simulink model "car_controller2222"  (R2022a)
settings: Solver=ode1be  StartTime=0.0  StopTime=1000  FixedStep=0.005  RelTol=1e-4  AbsTol=1e-4
libraries: simulink_extras x3, sim3dlib x1, uavsim3dlib x1
settings Model: Creator=Sebas  LastModifiedBy=maxpr
settings SolverCC: AutoScaleAbsTol=off  SolverJacobianMethodControl=SparsePerturbation  ZeroCrossControl=EnableAll  EnableFixedStepZeroCrossing=on
settings DebuggingCC: AlgebraicLoopMsg=none  UnconnectedInputMsg=warning  UnconnectedOutputMsg=warning  UnconnectedLineMsg=warning

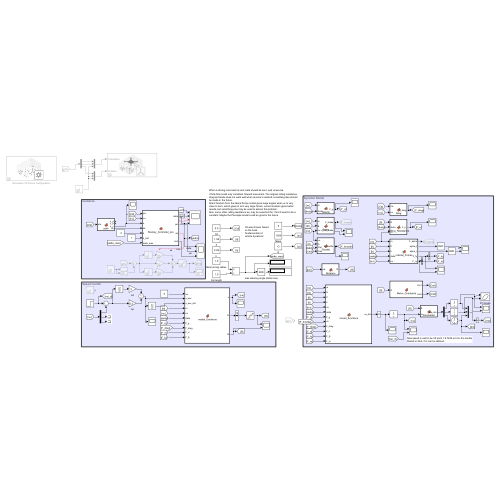
[thumbnail: Simulink's stored preview of the top-level diagram]
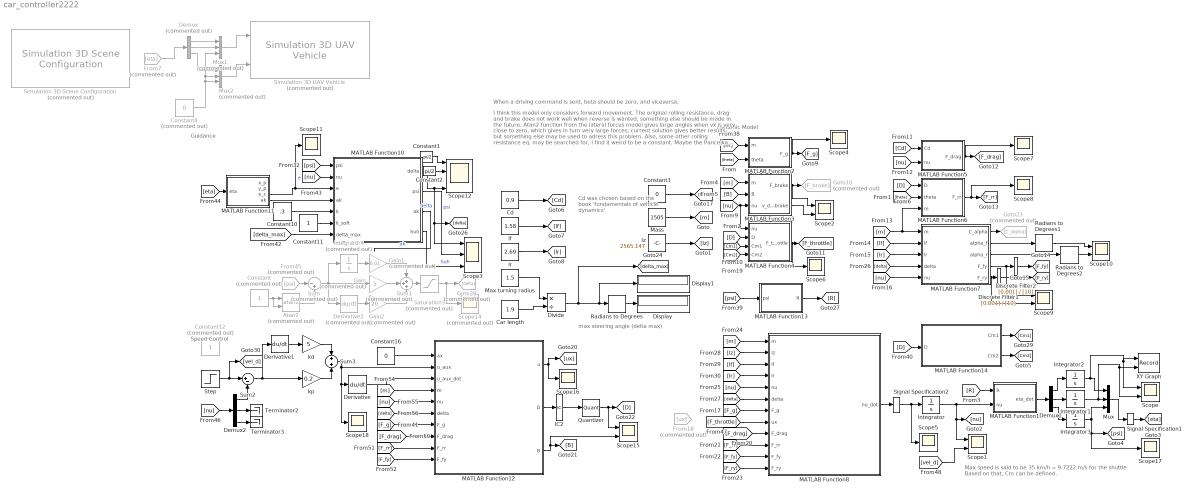
== system car_controller2222 ==
  note: Dynamic Model
  note: Guidance
  note: I think this model only considers forward movement. The original rolling resistance, drag and brake does not work well when reverse is wanted; something else should be made in the future.
      | Atan2 function from the lateral forces model gives large angles when vx is very close to zero, which gives in turn very large forces; current solution gives better results, but something else may be used to adress this problem.
      | Also, some other rolling resistance eq. may be searched for, I find it weird to be a constant. Maybe the Pancejka model could be good in the future.
  note: Max speed is said to be 35 km/h = 9.7222 m/s for the shuttle
      | Based on that, Cm can be defined.
  note: Cd was chosen based on the book 'fundamentals of vehicle dynamics'
  note: When a driving command is sent, beta should be zero, and viceversa.
  note: max steering angle (delta max)
  note: Speed Control
  Atan2 : Trigonometry  Commented=on  Operator=atan2
  Car length : Constant  Value=1.9
  Cd : Constant  Value=0.9
  Constant : Constant  Commented=on
  Constant1 : Constant  Value=-pi/2
  Constant10 : Constant  Value=.3
  Constant11 : Constant
  Constant12 : Constant  Commented=on
  Constant16 : Constant  Value=0
  Constant2 : Constant  Value=pi/2
  Constant3 : Constant  Value=0
  Constant4 : Constant  Commented=on  Value=0
  Demux : Demux  Commented=on  Outputs=3
  Demux1 : Demux  Outputs=3
  Demux2 : Demux  Outputs=3
  Derivative : Derivative
  Derivative1 : Derivative
  Derivative2 : Derivative  Commented=on
  Discrete Filter1 : DiscreteFilter  Numerator=[0.001]  Denominator=[10]
  Discrete Filter2 : DiscreteFilter  Numerator=[0.001]  Denominator=[10]
  Display : Display
  Display1 : Display
  Divide : Product  Inputs=*/
  From18 : From  Commented=on  GotoTag=ux
  From45 : From  Commented=on  GotoTag=psi
  From7 : From  Commented=on  GotoTag=eta
  Gain : Gain  Commented=on  Gain=5
  Gain1 : Gain  Commented=on  Gain=0.01
  Gain2 : Gain  Commented=on  Gain=20
  Goto10 : Goto  Commented=on  GotoTag=F_brake
  Goto23 : Goto  Commented=on  GotoTag=C_alpha
  Goto28 : Goto  Commented=on  GotoTag=delta
  IC2 : InitialCondition  Value=0
  Integrator : Integrator
  Integrator1 : Integrator
  Integrator2 : Integrator
  Integrator3 : Integrator  WrapState=on
  Integrator4 : Integrator  Commented=on
  Iz : Constant  Value=2565.147
  MATLAB Function1 : MATLAB Function  TreatAsAtomicUnit=on
  MATLAB Function10 : MATLAB Function  TreatAsAtomicUnit=on
  MATLAB Function11 : MATLAB Function  TreatAsAtomicUnit=on
  MATLAB Function12 : MATLAB Function  TreatAsAtomicUnit=on
  MATLAB Function13 : MATLAB Function  TreatAsAtomicUnit=on
  MATLAB Function14 : MATLAB Function  TreatAsAtomicUnit=on
  MATLAB Function2 : MATLAB Function  TreatAsAtomicUnit=on
  MATLAB Function3 : MATLAB Function  TreatAsAtomicUnit=on
  MATLAB Function4 : MATLAB Function  TreatAsAtomicUnit=on
  MATLAB Function5 : MATLAB Function  TreatAsAtomicUnit=on
  MATLAB Function6 : MATLAB Function  TreatAsAtomicUnit=on
  MATLAB Function7 : MATLAB Function  TreatAsAtomicUnit=on
  MATLAB Function8 : MATLAB Function  TreatAsAtomicUnit=on
  Mass : Constant  Value=1505
  Max turning radius : Constant  Value=1.5
  Mux : Mux  Inputs=3
  Mux1 : Mux  Commented=on  Inputs=3
  Mux2 : Mux  Commented=on  Inputs=3
  Quantizer : Quantizer  QuantizationInterval=1
  Radians to Degrees : simulink_extras/Transformations/Radians to Degrees
  Radians to Degrees1 : simulink_extras/Transformations/Radians to Degrees
  Radians to Degrees2 : simulink_extras/Transformations/Radians to Degrees
  Saturation3 : Saturate  Commented=on  UpperLimit=1.054  LowerLimit=-1.054
  Scope{,1..2,9..10,15} (6 alike) : Scope  NumInputPorts=2
  Scope{4..8,11,16..18} (9 alike) : Scope
  Scope12 : Scope  NumInputPorts=4
  Scope14 : Scope  Commented=on
  Scope3 : Scope  NumInputPorts=3
  Signal Specification1 : SignalSpecification
  Signal Specification2 : SignalSpecification  Dimensions=3
  Simulation 3D Scene Configuration : sim3dlib/Simulation 3D Scene Configuration  Priority=0  Commented=on  ProjectFormat=Default Scenes  SceneDesc=US city block  ProjectName=C:\Program Files\MATLAB\R2023a\toolbox\shared\sim3d_projects\automotive_project\UE4\WindowsNoEditor\VehicleSimulation.exe  ScenePath=/Game/Maps/USCityBlock  EnableOpenDRIVE=off  vehTagList={'Scene Origin';'SimulinkVehicle1'}  vehTag=Scene Origin  OpVisEn=off  Ts=.01  EnableWindow=on  EnableRemoteAccess=off  EnableWeather=off  SunAltitude=40.0  SunAzimuth=90  clouds=10  wind=1  fog=0  rain=0  sensorTag=MainCamera1  sensorId=1  sensorName=MainCamera1  mountLoc=Origin  offsetFlag=off  tmountOffset=[0, 0, 0]  rmountOffset=[0, 0, 0]  HorizontalResolution=1280  VerticalResolution=720  HorizontalFOV=60  mountPoint=[0 0 0]  mountOrientation=[0 0 0]  aMode=4  ID=1  GeoTrigger=Inactive
  Simulation 3D UAV Vehicle : uavsim3dlib/Simulation 3D UAV Vehicle  Priority=-1  Commented=on  Mesh=Quadrotor  MeshPath=/MathWorksUAVContent/UAVs/HexaRotorUAV/HexaRotor.HexaRotor  Color=Black  ActorName=SimulinkVehicle1  UseGlobalFrame=off  InitialTranslation=[0 0 0]  InitialRotation=[0 0 0]  InitialTranslationGlobal=[0 0 0]  InitialGeoOrigin=[0 0 0]  InitialRotationGlobal=[0 0 0]  SampleTime=-1  ActorType=SimulinkVehicle  ID=1  aMode=4  ActorTag=SimulinkVehicle1
  Step : Step  Time=0  Before=.5  After=.5  SampleTime=0
  Sum : Sum  Commented=on  Inputs=|-+
  Sum1 : Sum  Commented=on  Inputs=+++
  Sum2 : Sum  Inputs=|+-
  Sum3 : Sum
  Terminator2 : Terminator
  Terminator3 : Terminator
  XY Graph : Record  FileSettingsInternal="{\"entries\":[{\"content\":{\"excelSettings\":{\"content\":{},\"type\":\"Streamout.ExcelSettings\"}},\"type\":\"Streamout.FileSettingStorage\",\"uuid\":\"\"}],\"packageUris\":[\"http:\\/\\/schema.mathworks.com\\/mf0\\/streamout_blocks\\/R2020a\"],\"version\":\"1.0\"}"  Layout=[1 1]  SignalsInternal="{\"entries\":[{\"content\":{\"signals\":[{\"content\":{\"blockPath\":[],\"dimensions\":[1],\"domain\":\"\",\"lineColor\":\"#edb120\",\"plots\":[1],\"port\":1,\"signalID\":1411,\"signalName\":\"Integrator2\"},\"type\":\"RecordBlkView.Signal\",\"uuid\":\"\"},{\"content\":{\"blockPath\":[],\"dimensions\":[1],\"domain\":\"\",\"lineColor\":\"#7e2f8e\",\"plots\":[1],\"port\":2,\"signalID\":1414,\"signalName\":\"Integrator1\"},\"type\":\"RecordBlkView.Signal\",\"uuid\":\"\"}]},\"type\":\"RecordBlkView.InputSignals\",\"uuid\":\"\"}],\"packageUris\":[\"http:\\/\\/schema.mathworks.com\\/mf0\\/streamout_blocks\\/R2020a\"],\"version\":\"1.0\"}"  VisualizationBindings="{\"xyplotplugin\":{\"info\":[{\"series\":[{\"bindingParametersList\":[{\"parameter\":\"X-Axis\",\"signalID\":1411,\"signalName\":\"Integrator2\"},{\"parameter\":\"Y-Axis\",\"signalID\":1414,\"signalName\":\"Integrator1\"}],\"seriesID\":36310}],\"subplotID\":1}]}}"  CompatibilityTag=XY
  kd : Gain  Gain=5
  kp : Gain  Gain=0.2
  lf : Constant  Value=1.58
  lr : Constant  Value=2.69
  wires:
  Max turning radius/1 -> Divide/1
  Car length/1 -> Divide/2
  Radians to Degrees/1 -> Display/1
  Divide/1 -> Display1/1, Radians to Degrees/1, [delta_max]
  Iz/1 -> [Iz]
  Mass/1 -> [m]
  Cd/1 -> [Cd]
  lr/1 -> [lr]
  lf/1 -> [lf]
  [theta] -> MATLAB Function2/2(theta)
  [m] -> MATLAB Function3/1(m)
  [nu] -> MATLAB Function4/1(nu), MATLAB Function3/3(nu)
  [Cd] -> MATLAB Function5/1(Cd)
  [nu] -> MATLAB Function5/2(nu)
  [lf] -> MATLAB Function7/2(lf)
  [lr] -> MATLAB Function7/3(lr)
  [delta] -> MATLAB Function7/4(delta)
  [nu] -> MATLAB Function7/5(nu)
  MATLAB Function2/1(F_g) -> Scope4/1, [F_g]
  MATLAB Function3/1(F_brake) -> Scope2/1, Goto10/1
  MATLAB Function4/1(F_throttle) -> Scope6/1, [F_throttle]
  MATLAB Function5/1(F_drag) -> Scope7/1, [F_drag]
  MATLAB Function6/1(F_rr) -> Scope8/1, [F_rr]
  [F_g] -> MATLAB Function8/7(F_g)
  [F_drag] -> MATLAB Function8/9(F_drag)
  [F_rr] -> MATLAB Function8/10(F_rr)
  [F_fy] -> MATLAB Function8/11(F_fy)
  [F_ry] -> MATLAB Function8/12(F_ry)
  [m] -> MATLAB Function8/1(m)
  [nu] -> MATLAB Function8/5(nu)
  [delta] -> MATLAB Function8/6(delta)
  [Iz] -> MATLAB Function8/2(Iz)
  [lf] -> MATLAB Function8/3(lf)
  [lr] -> MATLAB Function8/4(lr)
  Integrator3/1 -> Scope17/1, [psi], Mux/3
  Demux1/3 -> Integrator3/1
  Integrator1/1 -> Scope/2, XY Graph/2, Mux/2
  Mux/1 -> Signal Specification1/1
  [R] -> MATLAB Function1/1(R)
  MATLAB Function1/1(eta_dot) -> Demux1/1
  Integrator/1 -> MATLAB Function1/2(nu), [nu], Scope1/1
  Integrator2/1 -> Scope/1, XY Graph/1, Mux/1
  Demux1/1 -> Integrator2/1
  Demux1/2 -> Integrator1/1
  [m] -> MATLAB Function2/1(m)
  [B] -> MATLAB Function3/2(B)
  MATLAB Function3/2(v_dot_brake) -> Scope2/2
  [m] -> MATLAB Function6/3(m), MATLAB Function7/1(m)
  Constant3/1 -> [theta]
  [theta] -> MATLAB Function6/2(theta)
  [D] -> MATLAB Function4/2(D)
  MATLAB Function7/3(alpha_r) -> Radians to Degrees2/1
  Radians to Degrees1/1 -> Scope10/1
  Radians to Degrees2/1 -> Scope10/2
  MATLAB Function7/1(C_alpha) -> Goto23/1
  Signal Specification1/1 -> [eta]
  MATLAB Function10/1(delta) -> Scope12/4, Scope3/1, [delta]  "delta"
  [eta] -> MATLAB Function11/1(eta)
  [psi] -> MATLAB Function10/1("psi ")
  MATLAB Function11/3(e_c) -> Scope11/1, MATLAB Function10/3(e)  "e"
  [nu] -> MATLAB Function10/2(nu)
  [delta_max] -> MATLAB Function10/7(delta_max)
  Constant11/1 -> MATLAB Function10/6(k_soft)
  Constant10/1 -> MATLAB Function10/5(k)
  Signal Specification2/1 -> Scope5/1, Integrator/1
  MATLAB Function7/2(alpha_f) -> Radians to Degrees1/1
  MATLAB Function7/5(F_ry) -> Scope9/2, Discrete Filter1/1
  MATLAB Function7/4(F_fy) -> Discrete Filter2/1, Scope9/1
  Discrete Filter1/1 -> [F_ry]
  Discrete Filter2/1 -> [F_fy]
  [psi] -> MATLAB Function13/1(psi)
  MATLAB Function13/1(R) -> [R]
  kp/1 -> Sum3/2
  Sum2/1 -> Derivative1/1, kp/1
  Demux2/1 -> Sum2/2
  Demux2/3 -> Terminator3/1
  Step/1 -> [vel_d], Sum2/1
  [nu] -> Demux2/1
  kd/1 -> Sum3/1
  Demux2/2 -> Terminator2/1
  Derivative1/1 -> kd/1
  Sum3/1 -> Scope18/1, Derivative/1, MATLAB Function12/2(u_aux)
  Constant16/1 -> MATLAB Function12/1(ax)
  MATLAB Function8/1(nu_dot) -> Signal Specification2/1
  [delta] -> MATLAB Function12/6(delta)
  [nu] -> MATLAB Function12/5(nu)
  [m] -> MATLAB Function12/4(m)
  [F_fy] -> MATLAB Function12/10(F_fy)
  [F_rr] -> MATLAB Function12/9(F_rr)
  [F_drag] -> MATLAB Function12/8(F_drag)
  [F_g] -> MATLAB Function12/7(F_g)
  MATLAB Function12/1(u) -> [ux], Scope16/1
  [F_throttle] -> MATLAB Function8/8(ux)
  Atan2/1 -> Sum/2
  Sum/1 -> Integrator4/1, Derivative2/1, Gain/1
  From45/1 -> Sum/1
  MATLAB Function12/3(B) -> Scope15/2, [B]
  MATLAB Function12/2(D) -> IC2/1
  Saturation3/1 -> Scope14/1, Goto28/1
  Sum1/1 -> Saturation3/1
  Derivative2/1 -> Gain2/1
  Constant/1 -> Atan2/2, Atan2/1
  Gain2/1 -> Sum1/3
  Gain/1 -> Sum1/2
  Integrator4/1 -> Gain1/1
  Gain1/1 -> Sum1/1
  Derivative/1 -> MATLAB Function12/3(u_aux_dot)
  MATLAB Function11/4(ak) -> MATLAB Function10/4("ak ")
  [D] -> MATLAB Function6/1(D)
  [Cm1] -> MATLAB Function4/3(Cm1)
  [Cm2] -> MATLAB Function4/4(Cm2)
  MATLAB Function14/2(Cm2) -> [Cm2]
  MATLAB Function14/1(Cm1) -> [Cm1]
  [D] -> MATLAB Function14/1(D)
  IC2/1 -> Quantizer/1
  Quantizer/1 -> Scope15/1, [D]
  [vel_d] -> Scope1/2
  Constant1/1 -> Scope12/1
  Constant2/1 -> Scope12/2
  ? -> Scope12/3
  MATLAB Function10/3(ak) -> ?  "ak"
  MATLAB Function10/2(psi) -> Scope3/2  "psi"
  MATLAB Function10/4(huh) -> Scope3/3  "huh"
  From7/1 -> Demux/1
  Demux/1 -> Mux1/1
  Demux/2 -> Mux1/2
  Constant4/1 -> Mux1/3, Mux2/2, Mux2/3
  Demux/3 -> Mux2/1
  Mux1/1 -> Simulation 3D UAV Vehicle/1
  Mux2/1 -> Simulation 3D UAV Vehicle/2

== matlab function car_controller2222/MATLAB Function8 ==
  data: m input; Iz input; lf input; lr input; nu input; delta input; F_g input; ux input; nu_dot output; F_drag input; F_rr input; F_fy input; F_ry input
function nu_dot = model_functions(m,Iz,lf,lr,nu,delta,F_g,ux, F_drag,F_rr,F_fy,F_ry)
    vx = nu(1);
    vy = nu(2);
    r = nu(3);
    
    fx =  -(F_drag + F_rr + F_g + F_fy*sin(delta) - m*vy*r)/m;
    fy = (F_ry + F_fy*cos(delta) - m*vx*r)/m;
    fz = (F_fy*lf*cos(delta) - F_ry*lr)/Iz;

    %ux = F_brake + F_throttle;
    uy = 0;
    uz = 0;

    gx = 1/m;
    gy = 0;
    gz = 0;

    f = [fx;fy;fz];
    g = [gx 0 0; 0 gy 0; 0 0 gz];
    u = [ux;uy;uz];

    nu_dot = f + g*u;
end

== matlab function car_controller2222/MATLAB Function10 ==
  data: psi input; nu input; e input; ak input; k input; k_soft input; delta_max input; delta output; psi output; ak output; huh output
function [delta, psi, ak, huh]= Stanley_Controller_pro(psi,nu,e,ak,k,k_soft,delta_max)
    v = norm(nu(1:2));
    %v = nu(1);

    %delta = -(psi - ak+ atan2(k*e,k_soft + v));
    delta = abs(psi-ak)+atan2(k*e,k_soft + v);
    huh = atan2(k*e,k_soft + v);

    if(delta > delta_max)
        delta = delta_max;
    elseif(delta < -delta_max)
        delta = -delta_max;
    end
    %delta = 0;
end

== matlab function car_controller2222/MATLAB Function11 ==
  data: x_p output; y_p output; e_c output; eta input; ak output
function [x_p,y_p,e_c,ak] = path(eta)
    path = [0 0;
             0.00001  100];

    e_x = path(2,1) - path(1,1);
    e_y = path(2,2) - path(1,2);

    ak = atan2(e_y,e_x);
    
    % Slope of path
    m1 = e_y/e_x;
    b = path(2,2) - m1*path(2,1);

    % Slope of normal line to the path
    m2 = -1/m1;
    c = eta(2) - m2*eta(1);

    % Obtain intersection point
    x_p = (c - b)/(m1 - m2);
    y_p = m1*x_p + b;
    %y_p = eta(2);
    %x_p = eta(1);


    % Crosstrack error in path frame
    e_c = -(eta(1)-x_p)*sin(ak) + (eta(2)-y_p)*cos(ak);

end

== matlab function car_controller2222/MATLAB Function12 ==
  data: ax input; u_aux input; u_aux_dot input; m input; nu input; delta input; F_g input; u output; F_drag input; F_rr input; F_fy input; D output size=1; B output size=1
function [u,D,B]= model_functions(ax,u_aux,u_aux_dot,m,nu,delta,F_g,F_drag,F_rr,F_fy)
    vx = nu(1);
    vy = nu(2);
    r = nu(3);

    B = 0;
    fx =  -(F_drag + F_rr + F_g + F_fy*sin(delta) - m*vy*r)/m;
    %gx = 1/m;
    u = m*(-fx + ax + u_aux);

    % Next condition was set so the vehicle does not move backwards when
    % the throttle force is less than the resistance
    if(F_rr >= u && vx < 0.01)
        u = F_rr;
    end

    x = roots([(0.0113-0.0028*vx) (0.4629*vx-2.0783) (134.067-22.399*vx) (-1038.7-u)]);
    y = x((real(x)>0&imag(x)==0));
    
    %disp("a")
    %disp(vx)
    %disp(u)
    %disp(y)
    D = real(y(1));
    
    if D>255
        D = 255;
    end

    %{
    if(u_aux_dot > 0)
        if(u > Cm)
            u = Cm;
        end
        D = u/Cm;
        B = 0;
    elseif(u_aux_dot < 0)
        
        B = u/m - 2.27 - 0.00535*vx;
        D = 0;
    end
    %}

end

== matlab function car_controller2222/MATLAB Function13 ==
  data: psi input; R output
function R = Rotation(psi)
    R = [cos(psi) sin(psi);
        -sin(psi) cos(psi)];
end

== matlab function car_controller2222/MATLAB Function14 ==
  data: D input; Cm1 output; Cm2 output
function [Cm1,Cm2]= Motor_Constants(D)

    Cm1 = 0.0113*D^2-2.1552*D+142.22;
    Cm2 = 0.0028*D^2-0.4629*D+22.399;

    %Cm1 = 120.78*exp(-0.013*D);
    %Cm2 = 16.762*exp(-0.019*D);

    %Cm1 = -0.7333*D + 102.59;
    %Cm2 = -0.1125*D + 12.631;

    %Cm1 = -43.63*log(D)+234.3;
    %Cm2 = -6.903*log(D)+33.706;

== matlab function car_controller2222/MATLAB Function1 ==
  data: R input; eta_dot output; nu input
function eta_dot = kinematics(R, nu)
    eta_dot = [0;0;nu(3)];
    eta_dot(1:2) = R*nu(1:2);
end

== matlab function car_controller2222/MATLAB Function2 ==
  data: m input; theta input; F_g output
function F_g = Gravity(m,theta)
    % theta : vehicle pitch angle
    g = 9.81;
    
    F_g = m*g*sin(theta);
end

== matlab function car_controller2222/MATLAB Function3 ==
  data: m input; B input; F_brake output; nu input; v_dot_brake output
function [F_brake,v_dot_brake]= Brake(m,B,nu)
    % B : pedal brake command (or position) [0, 1]
    
    vx = nu(1);
    % If this condition is not set, the simulation breaks as velocities
    % tend to infinity
    if(vx > 0)
        % I don't think the original model consider reverse motion nor
        % standstill situations.
        % Moreover, this model could lend excesive forces. A simple test
        % was made with initial longitudinal velocity of 3 m/s and the
        % brake force was -800 N; it could be important to analyze this
        % furthermore.
        % vdotbrake would be negative B>0.373
        v_dot_brake = min(0,2.27-6.12*B+0.00535*vx);
    else
        v_dot_brake = 0;
    end

    F_brake = m*v_dot_brake;
end

== matlab function car_controller2222/MATLAB Function4 ==
  data: nu input; F_throttle output; D input; Cm1 input; Cm2 input
function F_throttle = Throttle(nu,D,Cm1,Cm2)
    % Cm1 : motor model constant 1
    % Cm2 : motor model constant 2
    % D : throttle command (or position) [0, 255]

    vx = nu(1);

    offset = -0.0769*D^2 + 8.1533*D + 1038.7;
    %step 90 -> 1150
    %step 67 -> 1240
    %step 45 -> 1250

    if D>0
       F_throttle = (Cm1 - Cm2*vx)*D - offset;
    else
        F_throttle = 0;
    end

    %F_throttle = Cm*D;
    %F_throttle = Cm1 - Cm2*vx;

end

== matlab function car_controller2222/MATLAB Function5 ==
  data: Cd input; F_drag output; nu input
function F_drag = Drag(Cd,nu)
    % Cm : motor model constant
    % D : throttle command (or position) [0, 1]
    % ro : air density
    % A : transversal area
    % Cd : drag coefficient

    vx = nu(1);
    ro = 1.225;
    A = 3.426;
    
    F_drag = 0.5*ro*A*Cd*vx^2;
end

== matlab function car_controller2222/MATLAB Function6 ==
  data: D input; theta input; F_rr output; m input
function F_rr = Rolling_Resistance(D,theta,m)
    % fr : rolling resistance coefficient
    
    fr = 0.0776;
    %fr = 0.015; % For passenger cars, from fundamentals of vehicle dynamics book

    % This resistance force does does not consider standstill
    % situations. If the vehicle is at rest, the car moves backwards
    
    F_rr = m*9.81*fr*cos(theta); % From fundamentals of vehicle dynamics book
    
    offset = -0.0178*D^2 + 1.4012*D + 1018;
    %step 90 -> 1000
    %step 67 -> 1032
    %step 45 -> 1045

    %{
    if D == 0
        F_rr = F_rr - offset;
    end
    %}

    %F_rr = 1161.5 - 14.193*nu(1);

end

== matlab function car_controller2222/MATLAB Function7 ==
  data: C_alpha output; alpha_f output; alpha_r output; F_fy output; F_ry output; m input; lf input; lr input; delta input; nu input
function [C_alpha,alpha_f,alpha_r,F_fy,F_ry]= Lateral_Forces(m,lf,lr,delta,nu)
    % delta : steering angle
    % theta_vf : front tire velocity angle
    % theta_vr : rear tire velocity angle
    % C_alpha : tire cornering stiffness (assuming being equal for all tires)

    vx = nu(1);
    vy = nu(2);
    r = nu(3);

    % C alpha calculated from this webpage: https://www.mchenrysoftware.com/medit32/readme/msmac/default.htm?turl=examplestirecorneringstiffnesscalculation1.htm
    % Calculations made sense, as the Calpha of the Stanford Stanley car
    % are similar by being calculated with the same method
    C_alpha = m*9.81/2*0.165*57.2957; %N/rad

    alpha_f = atan2(vy + lf*r,vx) - delta;
    alpha_r = atan2(vy - lr*r,vx);

    if(vx > 0.01)
        % For some reason, atan2 was breaking the simulation in the integration
        % blocks using ode1 solver. By changing to ode14x or ode1b a better
        % response was acquired
        F_fy = -C_alpha*alpha_f;
        F_ry = -C_alpha*alpha_r;
    else
        F_fy = 0;
        F_ry = 0;
    end
end
